simulink model "integrator_filter_test"  (R2015b)
settings: Solver=VariableStepAuto  StartTime=0.0  StopTime=20  RelTol=1e-3
undefined symbols (not defined in the file): KFparam, std_R, Ts
settings Model: Creator=mgreiff  LastModifiedBy=mgreiff

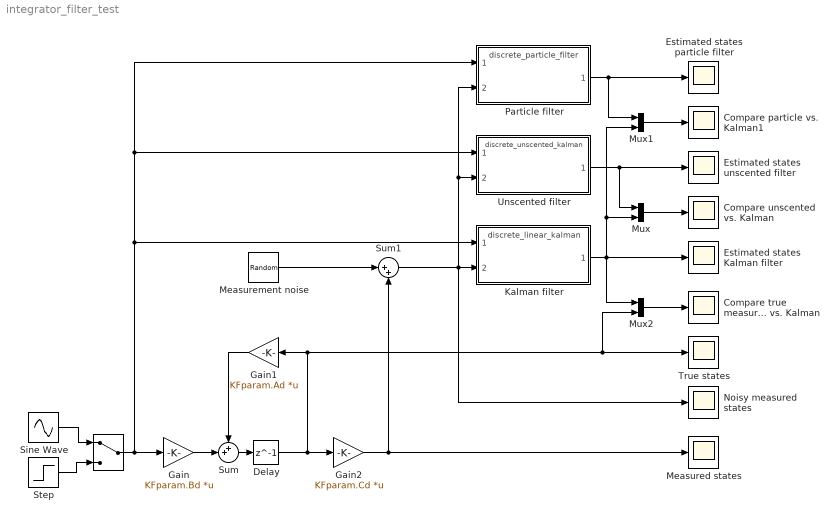
== system integrator_filter_test ==
  " " : ManualSwitch
  Compare particle vs. Kalman1 : Scope
  Compare true measurements vs. Kalman : Scope
  Compare unscented vs. Kalman : Scope
  Delay : Delay  DelayLength=1  InitialCondition=0  SampleTime=Ts
  Estimated states Kalman filter : Scope
  Estimated states particle filter : Scope
  Estimated states unscented filter : Scope
  Gain : Gain  Gain=KFparam.Bd  Multiplication=Matrix(K*u)
  Gain1 : Gain  Gain=KFparam.Ad  Multiplication=Matrix(K*u)
  Gain2 : Gain  Gain=KFparam.Cd  Multiplication=Matrix(K*u)
  Kalman filter : ModelReference  ModelNameDialog=discrete_linear_kalman.slx  SimulationMode=Normal  ModelReferenceVersion=1.88  CopyOfModelName=discrete_linear_kalman.slx
  Measured states : Scope
  Measurement noise : RandomNumber  Variance=std_R^2  SampleTime=Ts
  Mux : Mux  Inputs=2
  Mux1 : Mux  Inputs=2
  Mux2 : Mux  Inputs=2
  Noisy measured states : Scope
  Particle filter : ModelReference  ModelNameDialog=discrete_particle_filter.slx  SimulationMode=Normal  ModelReferenceVersion=1.15  CopyOfModelName=discrete_particle_filter.slx
  Sine Wave : Sin  SampleTime=0
  Step : Step  SampleTime=0
  Sum : Sum  Inputs=++|
  Sum1 : Sum  Inputs=|++
  True states : Scope
  Unscented filter : ModelReference  ModelNameDialog=discrete_unscented_kalman.slx  SimulationMode=Normal  ModelReferenceVersion=1.15  CopyOfModelName=discrete_unscented_kalman.slx
  wires:
  " "/1 -> Gain/1, Kalman filter/1, Particle filter/1, Unscented filter/1
  Delay/1 -> Gain2/1, True states/1, Mux2/2, Gain1/1
  Sum/1 -> Delay/1
  Gain1/1 -> Sum/1
  Gain2/1 -> Measured states/1, Sum1/2
  Kalman filter/1 -> Mux2/1, Estimated states Kalman filter/1, Mux1/2, Mux/2
  Sum1/1 -> Noisy measured states/1, Particle filter/2, Unscented filter/2, Kalman filter/2
  Measurement noise/1 -> Sum1/1
  Sine Wave/1 -> " "/1
  Step/1 -> " "/2
  Unscented filter/1 -> Mux/1, Estimated states unscented filter/1
  Particle filter/1 -> Mux1/1, Estimated states particle filter/1
  Mux/1 -> Compare unscented vs. Kalman/1
  Mux1/1 -> Compare particle vs. Kalman1/1
  Mux2/1 -> Compare true measurements vs. Kalman/1
  Gain/1 -> Sum/2
